simulink model "baseline_plant"  (R2025b)
settings: Solver=ode113  StartTime=0.0  StopTime=5801.231786  RelTol=1e-10  AbsTol=1e-10
InitFcn:
  | P = smallsat_params; ic = initial_state(P);
settings Model: Creator=USER  LastModifiedBy=USER

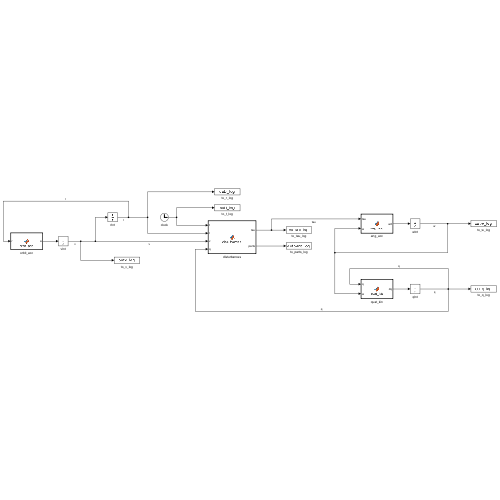
[thumbnail: Simulink's stored preview of the top-level diagram]
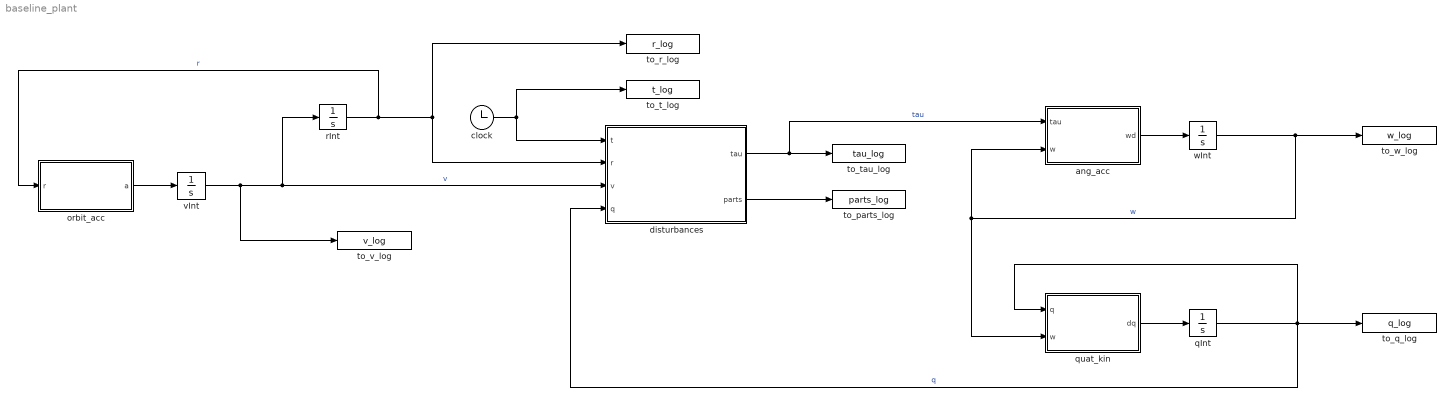
== system baseline_plant ==
  ang_acc : MATLAB Function  TreatAsAtomicUnit=on
  clock : Clock
  disturbances : MATLAB Function  TreatAsAtomicUnit=on
  orbit_acc : MATLAB Function  TreatAsAtomicUnit=on
  qInt : Integrator  InitialCondition=ic.q
  quat_kin : MATLAB Function  TreatAsAtomicUnit=on
  rInt : Integrator  InitialCondition=ic.r
  to_parts_log : ToWorkspace  VariableName=parts_log  SampleTime=10
  to_q_log : ToWorkspace  VariableName=q_log  SampleTime=10
  to_r_log : ToWorkspace  VariableName=r_log  SampleTime=10
  to_t_log : ToWorkspace  VariableName=t_log  SampleTime=10
  to_tau_log : ToWorkspace  VariableName=tau_log  SampleTime=10
  to_v_log : ToWorkspace  VariableName=v_log  SampleTime=10
  to_w_log : ToWorkspace  VariableName=w_log  SampleTime=10
  vInt : Integrator  InitialCondition=ic.v
  wInt : Integrator  InitialCondition=ic.w
  wires:
  rInt/1 -> orbit_acc/1(r), to_r_log/1, disturbances/2(r)  "r"
  orbit_acc/1(a) -> vInt/1
  vInt/1 -> to_v_log/1, rInt/1, disturbances/3(v)  "v"
  clock/1 -> to_t_log/1, disturbances/1(t)
  qInt/1 -> quat_kin/1(q), disturbances/4(q), to_q_log/1  "q"
  disturbances/1(tau) -> ang_acc/1(tau), to_tau_log/1  "tau"
  wInt/1 -> quat_kin/2(w), ang_acc/2(w), to_w_log/1  "w"
  ang_acc/1(wd) -> wInt/1
  quat_kin/1(dq) -> qInt/1
  disturbances/2(parts) -> to_parts_log/1

== matlab function baseline_plant/disturbances ==
  data: t input; tau output; r input; v input; q input; parts output; P parameter
function [tau, parts] = disturbances(t, r, v, q, P)
%#codegen
[tau, parts] = disturbance_block(t, r, v, q, P);
end

== matlab function baseline_plant/orbit_acc ==
  data: r input; a output; P parameter
function a = orbit_acc(r, P)
%#codegen
a = j2_accel(r, P);
end

== matlab function baseline_plant/ang_acc ==
  data: tau input; wd output; w input; P parameter
function wd = ang_acc(tau, w, P)
%#codegen
wd = P.inertia \ (tau - cross(w, P.inertia*w));
end

== matlab function baseline_plant/quat_kin ==
  data: q input; dq output; w input; P parameter
function dq = quat_kin(q, w, P)
%#codegen
dq = quat_rate(q, w);
end
